simulink model "dc5_iq_szinusz_elnyomas"  (R2013a)
settings: Solver=ode45  StartTime=0.0  StopTime=0.05  MaxStep=1e-7  RelTol=1e-3
undefined symbols (not defined in the file or in its folder): j
settings Model: Creator=balazs.varga  LastModifiedBy=balazs.varga

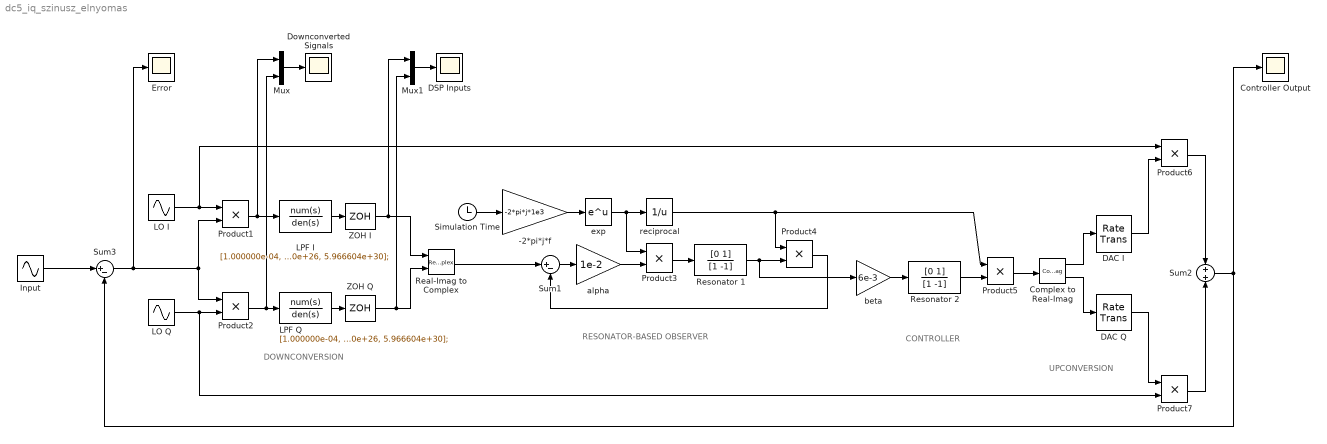
== system dc5_iq_szinusz_elnyomas ==
  note: UPCONVERSION
  note: CONTROLLER
  note: RESONATOR-BASED OBSERVER
  note: DOWNCONVERSION
  -2*pi*j*f : Gain  Gain=-2*pi*j*1e3  SampleTime=1/(64e3)
  Complex to Real-Imag : ComplexToRealImag  SampleTime=1/(64e3)
  Controller Output : Scope
  DAC I : RateTransition  OutPortSampleTimeOpt=Inherit
  DAC Q : RateTransition  OutPortSampleTimeOpt=Inherit
  DSP Inputs : Scope
      settings: YMin=0  YMax=0.5  SaveName=ScopeData3
  Downconverted Signals : Scope
      settings: YMin=0  YMax=0.5
  Error : Scope
      settings: YMin=-0.06  YMax=0.06  SaveName=ScopeData2
  Input : Sin  Frequency=2*pi*101e3  SampleTime=0
  LO I : Sin  Frequency=2*pi*100e3  Phase=pi/2  SampleTime=0
  LO Q : Sin  Frequency=2*pi*100e3  Phase=pi  SampleTime=0
  LPF I : TransferFcn  Numerator=[1.000000e-04, 3.637979e-16, 2.007439e+08, 6.803469e-04, 6.440612e+19, 1.408858e+08, 5.317742e+30];  Denominator=[1.000000e+00, 1.859046e+05, 8.074716e+10, 1.027346e+16, 1.700477e+21, 1.183100e+26, 5.966604e+30];
  LPF Q : TransferFcn  Numerator=[1.000000e-04, 3.637979e-16, 2.007439e+08, 6.803469e-04, 6.440612e+19, 1.408858e+08, 5.317742e+30];  Denominator=[1.000000e+00, 1.859046e+05, 8.074716e+10, 1.027346e+16, 1.700477e+21, 1.183100e+26, 5.966604e+30];
  Mux : Mux  Inputs=2
  Mux1 : Mux  Inputs=2
  Product{1..2,6..7} (4 alike) : Product
  Product3 : Product  SampleTime=1/(64e3)
  Product4 : Product  SampleTime=1/(64e3)
  Product5 : Product  SampleTime=1/(64e3)
  Real-Imag to Complex : RealImagToComplex  SampleTime=1/(64e3)
  Resonator 1 : DiscreteFilter  Numerator=[0 1]  Denominator=[1 -1]  SampleTime=1/(64e3)
  Resonator 2 : DiscreteFilter  Numerator=[0 1]  Denominator=[1 -1]  SampleTime=1/(64e3)
  Simulation Time : Clock
  Sum1 : Sum  Inputs=|+-  SampleTime=1/(64e3)
  Sum2 : Sum  Inputs=+|+
  Sum3 : Sum  Inputs=|+-
  ZOH I : ZeroOrderHold  SampleTime=1/(64e3)
  ZOH Q : ZeroOrderHold  SampleTime=1/(64e3)
  alpha : Gain  Gain=1e-2  SampleTime=1/(64e3)
  beta : Gain  Gain=6e-3  SampleTime=1/(64e3)
  "exp " : Math  SampleTime=1/(64e3)  SaturateOnIntegerOverflow=on
  reciprocal : Math  Operator=reciprocal  SampleTime=1/(64e3)  SaturateOnIntegerOverflow=on
  wires:
  LO I/1 -> Product6/1, Product1/1
  LO Q/1 -> Product7/2, Product2/2
  Product1/1 -> Mux/1, LPF I/1
  Product2/1 -> Mux/2, LPF Q/1
  LPF I/1 -> ZOH I/1
  LPF Q/1 -> ZOH Q/1
  ZOH I/1 -> Mux1/1, Real-Imag to Complex/1
  ZOH Q/1 -> Mux1/2, Real-Imag to Complex/2
  Product3/1 -> Resonator 1/1
  -2*pi*j*f/1 -> "exp "/1
  "exp "/1 -> reciprocal/1, Product3/1
  Resonator 1/1 -> Product4/2, beta/1
  reciprocal/1 -> Product5/1, Product4/1
  alpha/1 -> Product3/2
  Simulation Time/1 -> -2*pi*j*f/1
  Sum1/1 -> alpha/1
  Product4/1 -> Sum1/2
  Real-Imag to Complex/1 -> Sum1/1
  beta/1 -> Resonator 2/1
  Resonator 2/1 -> Product5/2
  Product5/1 -> Complex to Real-Imag/1
  Complex to Real-Imag/1 -> DAC I/1
  Complex to Real-Imag/2 -> DAC Q/1
  Product6/1 -> Sum2/1
  Product7/1 -> Sum2/2
  Input/1 -> Sum3/1
  Sum3/1 -> Error/1, Product1/2, Product2/1
  Sum2/1 -> Sum3/2, Controller Output/1
  DAC I/1 -> Product6/2
  DAC Q/1 -> Product7/1
  Mux/1 -> Downconverted Signals/1
  Mux1/1 -> DSP Inputs/1
